simulink model "task4_x_model"  (R2021b)
settings: Solver=FixedStepAuto  StartTime=0.0  StopTime=3  FixedStep=0.0001  RelTol=1e-3
settings Model: Creator=den  LastModifiedBy=den

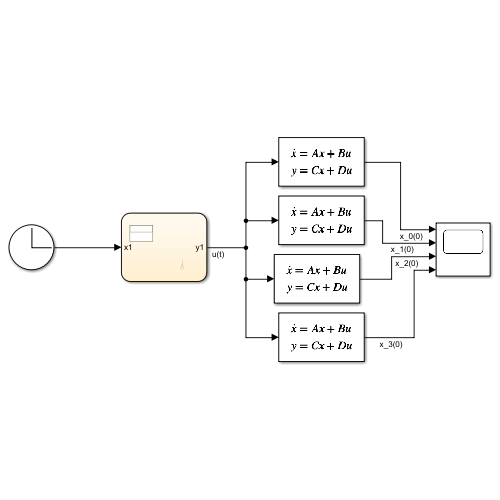
[thumbnail: Simulink's stored preview of the top-level diagram]
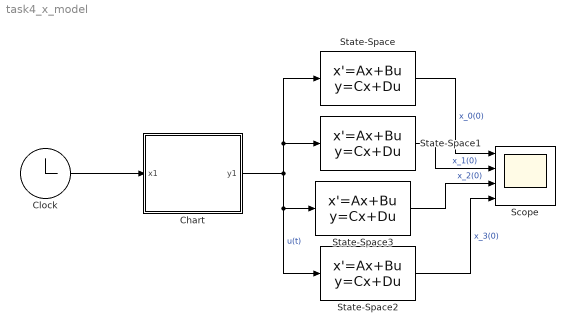
== system task4_x_model ==
  Chart : Stateflow chart  TreatAsAtomicUnit=on
  Clock : Clock
  Scope : Scope  NumInputPorts=4
  State-Space : StateSpace  A=[-7 9 1; -5 3 -3; 3 -7 -3]  B=[0; 0; 0]  C=[0 0 0; 0 0 0; 0 0 1]  D=[0; 0; 0]  InitialCondition=[-0.889, 0.778, -0.111]
  State-Space1 : StateSpace  A=[-7 9 1; -5 3 -3; 3 -7 -3]  B=[0; 0; 0]  C=[0 0 0; 0 0 0; 0 0 1]  D=[0; 0; 0]  InitialCondition=[0.111, 1.778, -1.111]
  State-Space2 : StateSpace  A=[-7 9 1; -5 3 -3; 3 -7 -3]  B=[0; 0; 0]  C=[0 0 0; 0 0 0; 0 0 1]  D=[0; 0; 0]  InitialCondition=[-1.889, -0.222, 0.889]
  State-Space3 : StateSpace  A=[-7 9 1; -5 3 -3; 3 -7 -3]  B=[0; 0; 0]  C=[0 0 0; 0 0 0; 0 0 1]  D=[0; 0; 0]  InitialCondition=[1.111, 2.778, -2.111]
  wires:
  Clock/1 -> Chart/1(x1)
  Chart/1(y1) -> State-Space3/1, State-Space2/1, State-Space1/1, State-Space/1  "u(t)"
  State-Space/1 -> Scope/1  "x_0(0)"
  State-Space1/1 -> Scope/2  "x_1(0)"
  State-Space2/1 -> Scope/4  "x_3(0)"
  State-Space3/1 -> Scope/3  "x_2(0)"

== matlab function task4_x_model/Chart ==
  data: x function_input; y function_output; x1 input; y1 output
function y = u(x)
    y = (-3 .* exp(-4 .* x)) .* cos(2 .* x) + (2 .* exp(-4  .* x)) .* sin(2 .* x);
end
